simulink library "Longitudinal_DrivingCycles"  (R2018b)
settings: Solver=VariableStepAuto  StartTime=0.0  StopTime=1477  RelTol=1e-3
undefined symbols (not defined in the file): cycle, DiscIntNeverNeededParam
settings Model: Creator=Tony  LastModifiedBy=ga69qig
settings SFSimCC: SimUseLocalCustomCode=off
settings RTWCC: RTWUseLocalCustomCode=off
settings CodeAppCC: StateflowObjectComments=on

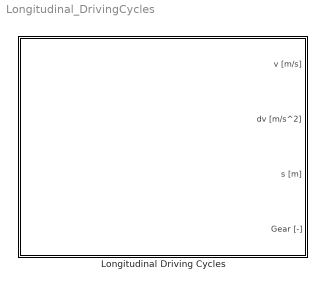
== system Longitudinal_DrivingCycles ==
  Longitudinal Driving Cycles : Subsystem  mask(SB){dcname=WLTP_class_2, dccircuits=1, dc_speed=cycle, dc_gear=[], LocalSampleTime=0}
      mask prompts: dcname "Choose Driving Cycle"; dccircuits "Number of Cycles"; dc_speed "Speed Vector [Nx2]"; dc_gear "Gear Vector [Nx2]"; LocalSampleTime "Local System Sample-Time [s]"
      mask help:
      | <Author> Tony Weiß, Alexander Koch, Benedikt Danquah based on Stefan Müller [1], Stephan Rohr [2]  </Author>
      | <Date> 06/04/2017 </Date>
      |
      | <Description> Allows to choose between 20 different driving cycles and gives the acceleration, speed, distance and gear for the corresponding time. Further option is to repeat the cycle. </Description>
      mask init:
      | GlobalSampleTime=CalcGlobalSampleTime(LocalSampleTime);
      | 
      | dc = init_driving_cycle (dcname, dccircuits, dc_speed,  dc_gear);
      mask Help:
      | <Parameters>
      | Choose Driving Cycle
      | 	<List> Europe_Artemis_Motorway; Europe_Artemis_Road; Europe_Artemis_Urban; Europe_City; Europe_EUDC; Europe_NEDC; Europe_UDC; Japan_10_15_MODE; Japan_10_MODE; Japan_10_MODE_3; Japan_11_MODE; Japan_11_MODE_4; Japan_15_MODE; USA_City_I; USA_City_II; USA_FTP_72; USA_FTP_75; USA_FTP_Highway; USA_NECC; WLTP_Class_1; WLTP_Class_2; WLTP_Class_3; Custom_Driving_Cycle
      | 
      | Number of Cycles [-]
      | 	<MIN: 1>
      | 
      | If Custom_Driving_Cycle is selected:
      | 
      | Speed Vector [1xN]
      | Time Vector [1xN]
      | Gear Vector [1xN]
      | 
      | with N ∈ {ℕ}
      | </Parameters>
      | 
      | <Inputs>
      | </Inputs>
      | 
      | <Outputs>
      | v [m/s]
      | dv [m/s^2]
      | s [m]
      | Gear [-]
      | </Outputs>
      | <Sources>
      | [1] S. Mueller, S. Rohr, W. Schmid, and M. Lienkamp, “Analysing the Influence of Driver Behaviour and Tuning Measures on Battery Aging and Residual Value of Electric Vehicles,” in Proc. EVS30 Symposium, Stuttgart, 2017, pp. 1–12.
      | [2] S. Rohr, “Technisch-wirtschaftliche Analyse des Zweitnutzungs- potentials von Lithium-Ionen-Traktionsbatterien,” Dissertation, Institute of Automotive Technology, Technical University Munich, Munich, 2018.
      | </Sources>
      mask TypeOptions dcname: EUROPE_ARTEMIS_MOTORWAY_130 | EUROPE_ARTEMIS_MOTORWAY_150 | EUROPE_ARTEMIS_ROAD | EUROPE_ARTEMIS_URBAN | EUROPE_City | EUROPE_EUDC | EUROPE_NEDC | EUROPE_UDC | JAPAN_10_15_MODE | JAPAN_10_MODE | JAPAN_10_MODE_3 | JAPAN_11_MODE | JAPAN_11_MODE_4 | JAPAN_15_MODE | USA_CITY_I | USA_CITY_II | USA_FTP_72 | USA_FTP_75 | USA_FTP_HIGHWAY | USA_NECC | WLTP_class_1 | WLTP_class_2 | WLTP_class_3 | Custom_Driving_Cycle
      mask Callback dcname:
      | var = get_param(gcb,'dcname');
      | maskObj = Simulink.Mask.get(gcb);
      | a = maskObj.Parameters;
      | 
      | off_params = ["dc_speed","dc_gear"];
      | 
      | for i = 1:length(a)
      |     for j = 1:length(off_params)
      |         if strcmp(maskObj.Parameters(i).Name,off_params(j))
      |             maskObj.Parameters(i).Visible = 'off';
      |             break;
      |         end
      |     end
      | end
      | 
      | if strcmp(var,'Custom_Driving_Cycle')
      |     for i = 1:length(a)
      |         maskObj.Parameters(i).Visible = 'on';
      |     end
      | end
      | 
      | %--------------------------------------------------------------------------
      | % Original callback
      | %--------------------------------------------------------------------------
      | %{
      | var = get_param(gcb,'dcname')
      | 
      | if strcmp(var,'Custom_Driving_Cycle')
      |     set_param(gcb,'MaskVisibilities',{'on';'on';'on';'on';'on'});
      | else
      |     set_param(gcb,'MaskVisibilities',{'on';'on';'off';'off';'off'});
      | end
      | %}
      mask DialogControl Container14 Prompt: Documentation:
      mask DialogControl DescHelpVar Prompt: %<MaskHelp>
      mask DialogControl Container4 Prompt: Sample Time
      mask Display:
      | port_label('output',1,'v [m/s]');
      | port_label('output',2,'dv [m/s^2]');
      | port_label('output',3,'s [m]');
      | port_label('output',4,'Gear [-]');
      | plot(dc.speedplot.Time,dc.speedplot.Data);

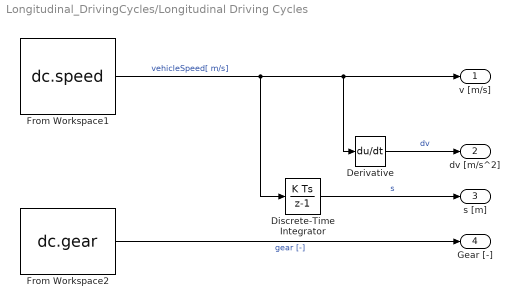
== system Longitudinal_DrivingCycles/Longitudinal Driving Cycles ==
  Derivative : Derivative
  Discrete-Time Integrator : DiscreteIntegrator  SampleTime=-1  ICPrevOutput=DiscIntNeverNeededParam  ICPrevScaledInput=DiscIntNeverNeededParam
  From Workspace1 : FromWorkspace  VariableName=dc.speed  SampleTime=LocalSampleTime
  From Workspace2 : FromWorkspace  VariableName=dc.gear  SampleTime=LocalSampleTime
  v [m/s] : Outport  SampleTime=GlobalSampleTime
  dv [m/s^2] : Outport  Port=2  SampleTime=GlobalSampleTime
  s [m] : Outport  Port=3  SampleTime=GlobalSampleTime
  Gear [-] : Outport  Port=4  SampleTime=GlobalSampleTime
  wires:
  From Workspace1/1 -> Discrete-Time Integrator/1, Derivative/1, v [m/s]/1  "vehicleSpeed[ m/s]"
  From Workspace2/1 -> Gear [-]/1  "gear [-]"
  Discrete-Time Integrator/1 -> s [m]/1  "s"
  Derivative/1 -> dv [m/s^2]/1  "dv"
